simulink model "up"  (Simulink 9.0)
settings: Solver=VariableStepAuto  StartTime=0.0  StopTime=10.0  RelTol=1e-3
values from neighbouring files (symbols this model uses):
  g = 9.80    (= 9.8)    [calcHinf.m]    (also in calcLQR.m; swingUp.m)
  I = 1/3*m*l^2    (= 0.00227083333333)    [calcHinf.m]    (also in calcLQR.m; swingUp.m)
  l = 0.25    [calcHinf.m]    (also in calcLQR.m; swingUp.m)
  m = 0.109    [calcHinf.m]    (also in calcLQR.m; swingUp.m)
undefined symbols (not defined in the file or in its folder): Klqr3
settings Model: Creator=Haotian  LastModifiedBy=Haotian
settings DataIOCC: SaveFormat=Dataset
settings OptimizationCC: LifeSpan=auto
settings DebuggingCC: UnderspecifiedInitializationDetection=Simplified  MergeDetectMultiDrivingBlocksExec=error  SFUnexpectedBacktrackingDiag=error  SFNoUnconditionalDefaultTransitionDiag=error  SFExecutionAtInitializationDiag=warning
settings HardwareCC: ProdBitPerPointer=64  ProdBitPerSizeT=64  ProdBitPerPtrDiffT=64  ProdLargestAtomicFloat=Float  ProdIntDivRoundTo=Zero  ProdEndianess=LittleEndian  ProdWordSize=64  ProdHWDeviceType=Intel->x86-64 (Windows64)
settings ModelReferenceCC: PropagateSignalLabelsOutOfModel=on
settings CodeAppCC: StateflowObjectComments=off
settings GRTTargetCC: TargetLangStandard=C99 (ISO)
settings ConfigComp: CovMetricSettings=dwe  CovHtmlReporting=off  CovSaveCumulativeToWorkspaceVar=off  CovSaveSingleToWorkspaceVar=off  CovExternalEMLEnable=on

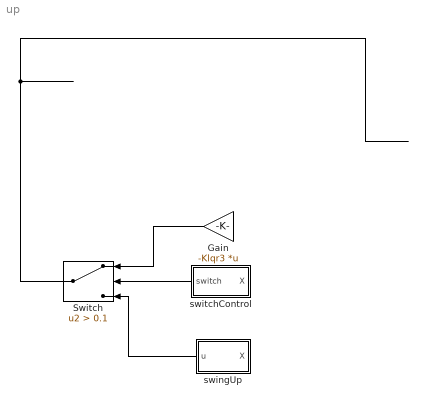
== system up ==
  Gain : Gain  Gain=-Klqr3  Multiplication=Matrix(K*u)
  Switch : Switch  Criteria=u2 > Threshold  Threshold=0.1
  swingUp : Subsystem
  switchControl : Subsystem
  wires:
  Switch/1 -> ?
  switchControl/1(switch) -> Switch/2
  Gain/1 -> Switch/1
  ? -> switchControl/1(X), swingUp/1(X), Gain/1
  swingUp/1(u) -> Switch/3

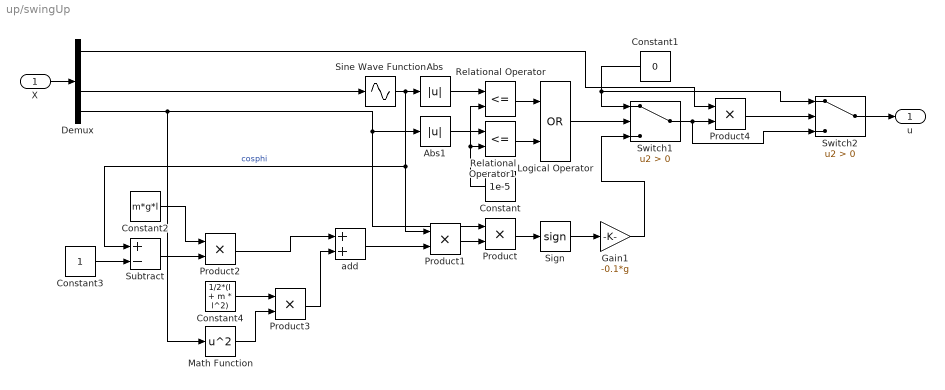
== system up/swingUp ==
  X : Inport
  Abs : Abs
  Abs1 : Abs
  Constant : Constant  Value=1e-5
  Constant1 : Constant  Value=0
  Constant2 : Constant  Value=m*g*l
  Constant3 : Constant
  Constant4 : Constant  Value=1/2*(I + m * l^2)
  Demux : Demux
  Gain1 : Gain  Gain=-0.1*g
  Logical Operator : Logic  Operator=OR  AllPortsSameDT=off  OutDataTypeStr=boolean
  Math Function : Math  Operator=square  SaturateOnIntegerOverflow=on
  Product{,1..4} (5 alike) : Product
  Relational Operator : RelationalOperator  Operator=<=  OutDataTypeStr=boolean  RndMeth=Simplest
  Relational Operator1 : RelationalOperator  Operator=<=  OutDataTypeStr=boolean  RndMeth=Simplest
  Sign : Signum
  Sine Wave Function : Sin  TimeSource=Use external signal  Phase=pi/2  SampleTime=0
  Subtract : Sum  Inputs=+-
  Switch1 : Switch  Criteria=u2 > Threshold
  Switch2 : Switch  Criteria=u2 > Threshold
  add : Sum
  u : Outport
  wires:
  Product2/1 -> add/1
  Constant3/1 -> Subtract/2
  Abs/1 -> Relational Operator/1
  Relational Operator1/1 -> Logical Operator/2
  Relational Operator/1 -> Logical Operator/1
  Constant/1 -> Relational Operator1/2, Relational Operator/2
  Subtract/1 -> Product2/2
  Product3/1 -> add/2
  Logical Operator/1 -> Switch1/2
  Abs1/1 -> Relational Operator1/1
  Product1/1 -> Product/2
  Product/1 -> Sign/1
  add/1 -> Product1/2
  Constant1/1 -> Switch2/1, Switch1/1
  Constant4/1 -> Product3/1
  Sign/1 -> Gain1/1
  Product4/1 -> Switch2/2
  Gain1/1 -> Switch1/3
  Demux/1 -> Product4/1
  Switch1/1 -> Switch2/3, Product4/2
  Demux/4 -> Math Function/1, Abs1/1, Product/1
  Sine Wave Function/1 -> Subtract/1, Product1/1, Abs/1  "cosphi"
  Demux/3 -> Sine Wave Function/1
  Switch2/1 -> u/1
  X/1 -> Demux/1
  Math Function/1 -> Product3/2
  Constant2/1 -> Product2/1

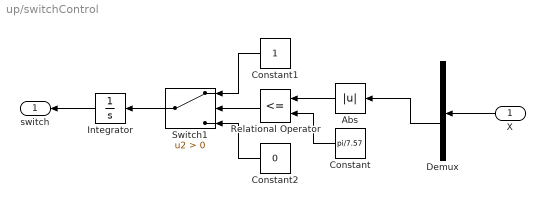
== system up/switchControl ==
  X : Inport
  Abs : Abs
  Constant : Constant  Value=pi/7.57
  Constant1 : Constant
  Constant2 : Constant  Value=0
  Demux : Demux
  Integrator : Integrator
  Relational Operator : RelationalOperator  Operator=<=  OutDataTypeStr=boolean  RndMeth=Simplest
  Switch1 : Switch  Criteria=u2 > Threshold
  switch : Outport
  wires:
  Constant2/1 -> Switch1/3
  Demux/3 -> Abs/1
  X/1 -> Demux/1
  Switch1/1 -> Integrator/1
  Constant/1 -> Relational Operator/2
  Constant1/1 -> Switch1/1
  Abs/1 -> Relational Operator/1
  Relational Operator/1 -> Switch1/2
  Integrator/1 -> switch/1
